simulink model "steeringwheel_ctrl"  (Simulink 6.4)
settings: Solver=FixedStepDiscrete  SolverMode=SingleTasking  StartTime=0  StopTime=inf  FixedStep=0.001  RelTol=1e-3
libraries: ecrobot_nxt_lib x7
CloseFcn:
  | rtwprivate ssgencode ModelCloseRequest TestBluetooth
settings Model: Creator=banno  LastModifiedBy=tchikama  ProdHWDeviceType=ARM7
settings DataIOCC: SaveOutput=off  SignalLogging=off  SaveTime=off
settings OptimizationCC: InlineParams=on  InlineInvariantSignals=on  RollThreshold=2  StateBitsets=on  DataBitsets=on  UseTempVars=on  InitFltsAndDblsToZero=off  NoFixptDivByZeroProtection=on  EfficientFloat2IntCast=on  OptimizeModelRefInitCode=on  LifeSpan=1
settings DebuggingCC: ConsistencyChecking=warning  SignalInfNanChecking=warning  ReadBeforeWriteMsg=DisableAll  WriteAfterWriteMsg=DisableAll  WriteAfterReadMsg=DisableAll  AlgebraicLoopMsg=error  CheckExecutionContextPreStartOutputMsg=on  CheckExecutionContextRuntimeOutputMsg=on  SolverPrmCheckMsg=none  SingleTaskRateTransMsg=warning  TasksWithSamePriorityMsg=none  IntegerOverflowMsg=error  ParameterPrecisionLossMsg=none  UnconnectedInputMsg=error  UnconnectedOutputMsg=error  UnconnectedLineMsg=error  UniqueDataStoreMsg=error  BusObjectLabelMismatch=error  RootOutportRequireBusObject=error  ModelReferenceIOMsg=warning  ModelReferenceVersionMismatchMessage=warning  ModelReferenceIOMismatchMessage=warning
settings HardwareCC: ProdIntDivRoundTo=Zero  ProdEndianess=LittleEndian  ProdHWDeviceType=ARM7  TargetHWDeviceType=32-bit Generic
settings ModelReferenceCC: ModelReferenceNumInstancesAllowed=Single
settings RTWCC: SystemTargetFile=ert.tlc  GenCodeOnly=on  GenerateMakefile=off  TemplateMakefile=ert_default_tmf  Description=Real-Time Workshop Embedded Coder (no auto configuration)  GenerateReport=on  RTWVerbose=off  ProcessScript=ert_make_rtw_hook  IncludeHyperlinkInReport=on  LaunchReport=on
settings CodeAppCC: ForceParamTrailComments=on  IgnoreCustomStorageClasses=off  SFDataObjDesc=on  PrefixModelToSubsysFcnNames=off  CustomSymbolStrGlobalVar=rt$N$M  CustomSymbolStrType=$N$M  CustomSymbolStrFcn=$N$M$F  CustomSymbolStrMacro=$N$M  InsertBlockDesc=on
settings ERTTargetCC: TargetFcnLib=ansi_tfl_tmw.mat  GenFloatMathFcnCalls=GNU  IncludeMdlTerminateFcn=off  SuppressErrorStatus=on  IncludeERTFirstTime=on  SupportAbsoluteTime=off  SupportNonFinite=off  SupportComplex=off  InlinedParameterPlacement=NonHierarchical  RootIOFormat=Structure reference  ERTCustomFileTemplate=example_file_process.tlc  InitialValueSource=Model

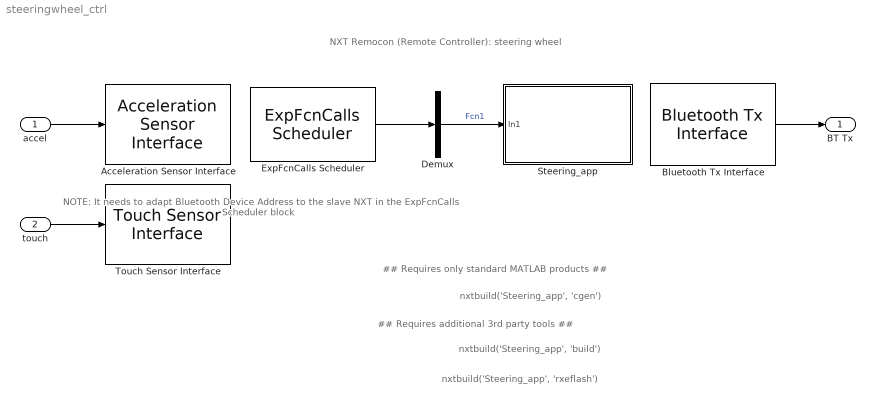
== system steeringwheel_ctrl ==
  note: nxtbuild('Steering_app', 'build')
  note: nxtbuild('Steering_app', 'rxeflash')
  note: nxtbuild('Steering_app', 'cgen')
  note: ## Requires only standard MATLAB products ##
  note: ## Requires additional 3rd party tools ##
  note: NOTE: It needs to adapt Bluetooth Device Address to the slave NXT
      | in the ExpFcnCalls Scheduler block
  note: NXT Remocon (Remote Controller): steering wheel
  accel : Inport  DataType=int16
  touch : Inport  Port=2  OutDataType=fixdt(1,16,0)  OutScaling=[]
  Acceleration Sensor Interface : ecrobot_nxt_lib/Acceleration Sensor Interface  SystemSampleTime=-1  ip=S1
  Bluetooth Tx Interface : ecrobot_nxt_lib/Bluetooth Tx Interface  SystemSampleTime=-1
  Demux : Demux  Outputs=1
  ExpFcnCalls Scheduler : ecrobot_nxt_lib/ExpFcnCalls Scheduler  Priority=1  fcname='Fcn1'  fctrigger=[10]  ts=0.001  platform=OSEK  stacksize=[512]  bd_mode=Master  bd_addr='00', '16', '53', '04', 'F1', 'B3', '00'
  Steering_app : Subsystem
      mask Display: image(imread('steeringwheel_ctrl.JPG'))
  Touch Sensor Interface : ecrobot_nxt_lib/Touch Sensor Interface  SystemSampleTime=-1  ip=S2
  BT Tx : Outport
  wires:
  ExpFcnCalls Scheduler/1 -> Demux/1
  Demux/1 -> Steering_app/1(In1)  "Fcn1"
  Bluetooth Tx Interface/1 -> BT Tx/1
  accel/1 -> Acceleration Sensor Interface/1
  touch/1 -> Touch Sensor Interface/1

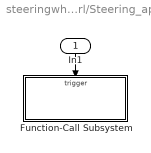
== system steeringwheel_ctrl/Steering_app ==
  In1 : Inport  Orientation=down
  Function-Call Subsystem : Subsystem  TreatAsAtomicUnit=on
  wires:
  In1/1 -> Function-Call Subsystem/Trigger

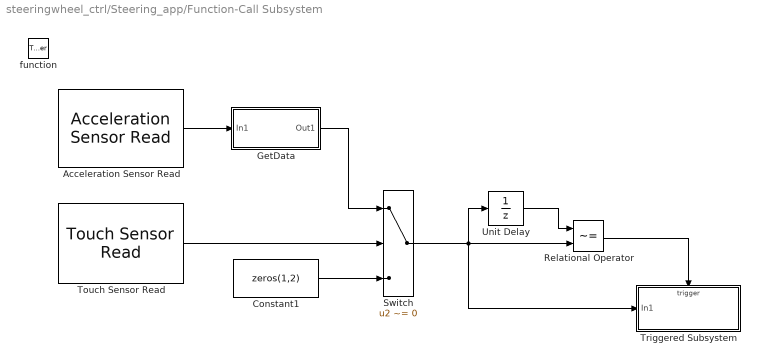
== system steeringwheel_ctrl/Steering_app/Function-Call Subsystem ==
  function : TriggerPort  TriggerType=function-call
  Acceleration Sensor Read : ecrobot_nxt_lib/Acceleration Sensor Read  ip=S1
  Constant1 : Constant  Value=zeros(1,2)  OutDataTypeMode=uint8  OutDataType=sfix(16)  ConRadixGroup=Use specified scaling  OutScaling=2^0  SampleTime=-1  FramePeriod=inf
  GetData : Subsystem
  Relational Operator : RelationalOperator  Operator=~=  LogicOutDataTypeMode=Boolean
  Switch : Switch  Criteria=u2 ~= 0
  Touch Sensor Read : ecrobot_nxt_lib/Touch Sensor Read  SystemSampleTime=-1  ip=S2
  Triggered Subsystem : Subsystem  TreatAsAtomicUnit=on
  Unit Delay : UnitDelay  SampleTime=-1
  wires:
  Touch Sensor Read/1 -> Switch/2
  Constant1/1 -> Switch/3
  Acceleration Sensor Read/1 -> GetData/1(In1)
  GetData/1(Out1) -> Switch/1
  Relational Operator/1 -> Triggered Subsystem/Trigger
  Unit Delay/1 -> Relational Operator/1
  Switch/1 -> Triggered Subsystem/1(In1), Unit Delay/1, Relational Operator/2

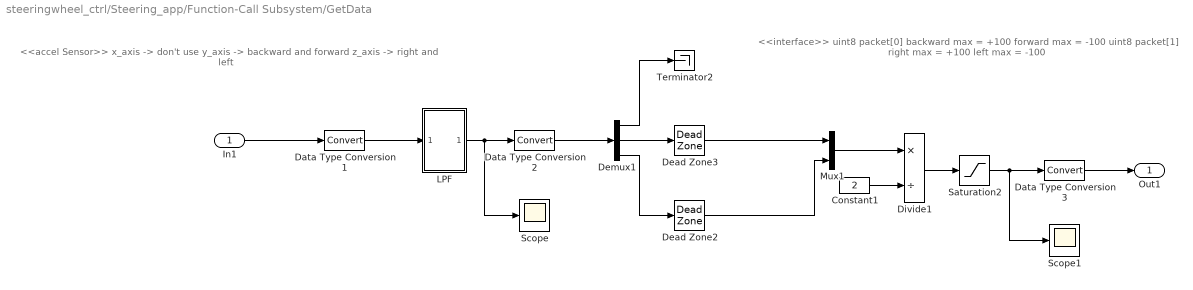
== system steeringwheel_ctrl/Steering_app/Function-Call Subsystem/GetData ==
  note: <<accel Sensor>>
      | x_axis -> don't use
      | y_axis -> backward and forward
      | z_axis -> right and left
  note: <<interface>>
      | uint8 packet[0]
      |   backward max = +100
      |   forward max = -100
      | uint8 packet[1]
      |   right max = +100
      |   left max = -100
  In1 : Inport  OutDataType=fixdt(1,16,0)  OutScaling=[]
  Constant1 : Constant  Value=2  OutDataType=sfix(16)  ConRadixGroup=Use specified scaling  OutScaling=2^0  SampleTime=inf  FramePeriod=inf
  Data Type Conversion1 : DataTypeConversion  OutDataTypeMode=single
      settings: AttributesFormatString=Round = %<RndMeth>
  Data Type Conversion2 : DataTypeConversion  OutDataTypeMode=int16  RndMeth=Simplest
      settings: AttributesFormatString=Round = %<RndMeth>
  Data Type Conversion3 : DataTypeConversion  OutDataTypeMode=uint8  RndMeth=Simplest
      settings: AttributesFormatString=Round = %<RndMeth>
  Dead Zone2 : DeadZone  LowerValue=-20  UpperValue=20  SaturateOnIntegerOverflow=on
  Dead Zone3 : DeadZone  LowerValue=-40  UpperValue=40  SaturateOnIntegerOverflow=on
  Demux1 : Demux  Outputs=3
  Divide1 : Product  Inputs=*/  OutScaling=2^-10  RndMeth=Simplest
  LPF : Subsystem
  Mux1 : Mux  Inputs=2
  Saturation2 : Saturate  UpperLimit=70  LowerLimit=-70  LinearizeAsGain=off
  Scope : Scope
      settings: TimeRange=20  YMin=-300  YMax=300
  Scope1 : Scope
      settings: TimeRange=20  YMin=-100  YMax=100
  Terminator2 : Terminator
  Out1 : Outport  OutDataType=fixdt(1,16,0)  OutScaling=[]
  wires:
  Data Type Conversion1/1 -> LPF/1(In1)
  LPF/1(Out1) -> Data Type Conversion2/1, Scope/1
  In1/1 -> Data Type Conversion1/1
  Dead Zone3/1 -> Mux1/1
  Demux1/1 -> Terminator2/1
  Demux1/2 -> Dead Zone3/1
  Demux1/3 -> Dead Zone2/1
  Data Type Conversion2/1 -> Demux1/1
  Saturation2/1 -> Data Type Conversion3/1, Scope1/1
  Data Type Conversion3/1 -> Out1/1
  Dead Zone2/1 -> Mux1/2
  Mux1/1 -> Divide1/1
  Constant1/1 -> Divide1/2
  Divide1/1 -> Saturation2/1

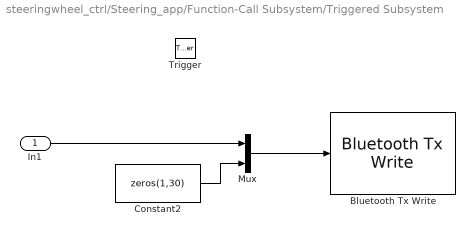
== system steeringwheel_ctrl/Steering_app/Function-Call Subsystem/Triggered Subsystem ==
  In1 : Inport
  Trigger : TriggerPort  TriggerType=either
  Bluetooth Tx Write : ecrobot_nxt_lib/Bluetooth Tx Write
  Constant2 : Constant  Value=zeros(1,30)  OutDataTypeMode=uint8  OutDataType=sfix(16)  ConRadixGroup=Use specified scaling  OutScaling=2^0  SampleTime=-1  FramePeriod=inf
  Mux : Mux  Inputs=2
  wires:
  Mux/1 -> Bluetooth Tx Write/1
  Constant2/1 -> Mux/2
  In1/1 -> Mux/1

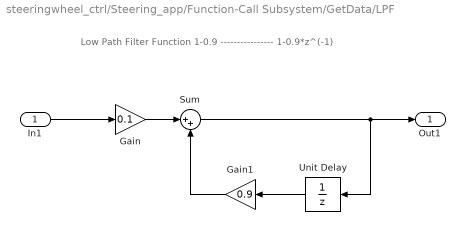
== system steeringwheel_ctrl/Steering_app/Function-Call Subsystem/GetData/LPF ==
  note: Low Path Filter Function
      |       1-0.9
      |          ----------------
      |          1-0.9*z^(-1)
  In1 : Inport
  Gain : Gain  Gain=0.1
  Gain1 : Gain  Orientation=left  Gain=0.9
  Sum : Sum  Inputs=|++
  Unit Delay : UnitDelay  Orientation=left  SampleTime=-1
  Out1 : Outport
  wires:
  Gain1/1 -> Sum/2
  Sum/1 -> Unit Delay/1, Out1/1
  Gain/1 -> Sum/1
  Unit Delay/1 -> Gain1/1
  In1/1 -> Gain/1
